simulink model "IEEE24bus"  (R2019b)
settings: Solver=VariableStepAuto  StartTime=0.0  StopTime=100  RelTol=1e-3
values from neighbouring files (symbols this model uses):
  C_b = 1/(w_b*Z_b)    (= 5.01433343075e-06)    [IEEE24_bus.m]
  Exc = [ 011	0	 200	0.02	1.12   0.5   0	0       0       0       0       0 ... (first row only)    [IEEE24_bus.m]
  G_data = [ 011	15.8 138	2.8	0.2     2.7	1.5     0.3     7.5     0.25	0.04	0.85	0.85	0.25	0.12	0 ... (first row only)    [IEEE24_bus.m]
  H011 = 4    [IEEE24_bus.m]
  H012 = 4    [IEEE24_bus.m]
  H013 = 4    [IEEE24_bus.m]
  H021 = 4    [IEEE24_bus.m]
  H022 = 4    [IEEE24_bus.m]
  H023 = 4    [IEEE24_bus.m]
  H024 = 4    [IEEE24_bus.m]
  H025 = 4    [IEEE24_bus.m]
  H026 = 4    [IEEE24_bus.m]
  H131 = 4    [IEEE24_bus.m]
  H132 = 4    [IEEE24_bus.m]
  H133 = 4    [IEEE24_bus.m]
  H134 = 4    [IEEE24_bus.m]
  H135 = 4    [IEEE24_bus.m]
  H151 = 4    [IEEE24_bus.m]
  H152 = 4    [IEEE24_bus.m]
  H153 = 4    [IEEE24_bus.m]
  H154 = 4    [IEEE24_bus.m]
  H161 = 4    [IEEE24_bus.m]
  H181 = 3.25    [IEEE24_bus.m]
  H211 = 4    [IEEE24_bus.m]
  H212 = 4    [IEEE24_bus.m]
  H213 = 4    [IEEE24_bus.m]
  H215 = 4    [IEEE24_bus.m]
  H216 = 4    [IEEE24_bus.m]
  H221 = 3.25    [IEEE24_bus.m]
  H231 = 4    [IEEE24_bus.m]
  H232 = 4    [IEEE24_bus.m]
  H233 = 4    [IEEE24_bus.m]
  H234 = 4    [IEEE24_bus.m]
  H235 = 4    [IEEE24_bus.m]
  L_b = Z_b/w_b    (= 1.40321608159)    [IEEE24_bus.m]
  PSSMODEL = 1    [IEEE24_bus.m]    (also in IEEE24bus_simplified_benchmark.m)
  Z_b = (V_b^2)/S_b    (= 529)    [IEEE24_bus.m]
undefined symbols (not defined in the file or in its folder): D1, Delta
libraries: powerlib x258, sps_avr x33, microgridLibrary x6
(part 4 of 6)

== system IEEE24bus/151 ==
  151 : powerlib/Machines/Synchronous Machine pu Standard  PresetModel=No  MechanicalLoad=Mechanical power Pm  ShowDetailedParameters=on  RotorType=Round  Units=per unit standard parameters  MeasurementBus=off  NominalParameters="[G_data(16,2)*1E6  G_data(16,3)*1E3  60]"  Reactances1=[G_data(16,6),G_data(16,8),G_data(16,10),G_data(16,7),G_data(16,12),G_data(16,14),G_data(16,5)]  Reactances2=[G_data(6,6),G_data(6,8),G_data(6,10),G_data(6,7),G_data(6,12),G_data(6,14),G_data(6,5)]  dAxisTimeConstants=Open-circuit  qAxisTimeConstants=Open-circuit  TimeConstants1="[G_data(6,9)  G_data(6,11)  G_data(6,13)  G_data(6,15)]"  TimeConstants2="[G_data(16,9)  G_data(16,11)  G_data(16,13)  G_data(16,15)]"  TimeConstants3="[  5.9  0.033  0.023  ]"  TimeConstants4=[ 8.0, 0.03, 0.3371, 0.0295 ]  TimeConstants5=[ 1.01, 0.053, 0.1 ]  TimeConstants6=[ 1.3201, 0.023, 1.0, 0.07 ]  TimeConstants7="[  1.01  0.053  0.051266  ]"  TimeConstants8=[ 1.3201, 0.0231, 0.3371, 0.0295 ]  StatorResistance=0  Mechanical="[ H151 0  4 ]"  PolePairs=4  InitialConditions=[0 -49.0871 0.832503 0.832503 0.832503 -10.6328 -130.633 109.367 2.39024]  SetSaturation=off  Saturation=[0.6404,0.7127,0.8441,0.9214,0.9956,1.082,1.19,1.316,1.457;0.7,0.7698,0.8872,0.9466,0.9969,1.046,1.1,1.151,1.201]  LoadFlowParameters=[1 3330000000 20000 0 0]  TsPowergui=0  TsBlock=-1  IterativeModel=Forward Euler  IterativeDiscreteModel=Trapezoidal non iterative  BusType=PV  Pref=G_data(16,2)*1e6  Qref=0  Qmin=-inf  Qmax=inf  PLF=0  QLF=0
      settings: SourceProductName=Simscape Power Systems
  AC4A Excitation System 151 : sps_avr/AC4A Excitation System  Tr=Exc(16,2)  KaTa="[Exc(16,3)   Exc(16,4)]"  VIminmax=[-10 10]  VRminmax=[-4.53 5.64]  TbTc="[Exc(16,5)  Exc(16,6)]"  Kc=0  v0=[1 2.3902]  TsBlock=0
      link override Model/Low Pass Filter 1//(Tr.s+1): Y0=Vt0  U0=Vt0
      settings: SourceProductName=Simscape Power Systems  SourceProductBaseCode=PS
  Bus Selector1 : BusSelector  OutputSignals="Mechanical.Rotor speed  wm  (pu),Output active power   Peo (pu),Mechanical.Rotor speed deviation  dw (pu),Mechanical.Rotor angle deviation  d_theta (rad),Mechanical.Rotor mechanical angle  theta (deg),dq0 components.Stator voltage  vd (pu),dq0 components.Stator voltage  vq (pu),dq0 components.Field current  ifd (pu),Output reactive power  Qeo (pu)"
  Complex to Magnitude-Angle : ComplexToMagnitudeAngle  Output=Magnitude
  "Delta Pa PSS 151 " : powerlib/Machines/Generic Power System Stabilizer  Tsensor=15e-3  K=2.5*1.25  Twashout=1  Tleadlag1=[60e-3 1]  Tleadlag2=[0 0]  VSlimits=[-0.15 0.15]  Vinit=0  Plot_On=off  MagdB_On=on  FreqRange=logspace(-2,2,500)
      settings: SourceProductName=Simscape Power Systems  SourceProductBaseCode=PS
  "Delta w PSS (Kundur) 151 " : powerlib/Machines/Generic Power System Stabilizer  Tsensor=15e-3  K=30  Twashout=10  Tleadlag1=[50e-3 20e-3]  Tleadlag2=[3 5.4]  VSlimits=[-0.15 0.15]  Vinit=0  Plot_On=off  MagdB_On=on  FreqRange=logspace(-2,2,500)
      settings: SourceProductName=Simscape Power Systems  SourceProductBaseCode=PS
  MB-PSS  151 : powerlib/Machines/Multi-Band Power System Stabilizer  OperationMode=Simplified settings  Kg=1  GL=[0.1 10]  GI="[1  10]"  GH="[13  120]"  GLd=[66 66 9.4]  TcLF=[1.667 2 0 0 0 0 2 2.4 0 0 0 0 1 1]  GId=[66 66 47.6]  TcIF=[1 1 0.25 0.3 0 0 1 1 0.3 0.36 0 0 0 0]  GHd=[66 66 233]  TcHF="[0.01 0.012 0 0 0 0  0.012 0.0144 0 0 0 0 1 1]"  LIM=[.075 .15 .15 .15]  Plot_On=off  MagdB_On=off  FreqRange=logspace(-2,2,500)
      settings: SourceProductName=Simscape Power Systems  SourceProductBaseCode=PS
  Multiport Switch1 : MultiPortSwitch  Inputs=4  InputSameDT=on
  PSS model3 : Constant  Value=0
  PSS model4 : Constant
  Pref : Constant
  Real-Imag to Complex : RealImagToComplex
  STG 151 : powerlib/Machines/Steam Turbine and Governor  gentype=Tandem-compound (single mass)  reg1="[ 1  0.05    0 ]"  reg2="[ 0.001  0.15 ]"  reg3="[ -0.1  0.1  0  4.496 ]"  N=3600  turb1="[ 0  10   3.3   0.5   ]"  turb2="[   0   0.36    0.36   0.28   ]"  HA="[ 0.046  1.430  1.465   0.192 ]"  KA="[ 90.44  53.88  64.59   62.94  ]"  DA="[ 0.0115  0.3575  0.3663   0.0137  ]"  ini1=0.9  ini2=[0.779316,-31.4247]
      settings: SourceProductName=Simscape Power Systems  SourceProductBaseCode=PS
  Sum2 : Sum  SaturateOnIntegerOverflow=on  InputSameDT=on  OutDataTypeStr=Inherit: Same as first input
  Sum3 : Sum  Inputs=-+  SaturateOnIntegerOverflow=on  InputSameDT=on  OutDataTypeStr=Inherit: Same as first input
  Terminator1 : Terminator
  Terminator2 : Terminator
  Terminator3 : Terminator
  Vref151 : Constant
  wref : Constant
  A : PMIOPort  Side=Left
  B : PMIOPort  Port=2  Side=Left
  C : PMIOPort  Port=3  Side=Left
  tag scope: EFD151=global, Pa151=global, Pe151=global, Pm151=global, Q151=global, Vt151=global, d_theta151=global, pss151=global, theta151=global, w151=global
  wires:
  Bus Selector1/7 -> Real-Imag to Complex/2  "<Stator voltage  vq (pu)>"
  Bus Selector1/6 -> Real-Imag to Complex/1  "<Stator voltage  vd (pu)>"
  wref/1 -> STG 151/1
  Vref151/1 -> AC4A Excitation System 151/1
  Bus Selector1/4 -> [d_theta151], STG 151/4  "<Rotor angle deviation  d_theta (rad)>"
  151/1 -> Bus Selector1/1, [M151]
  Bus Selector1/1 -> [w151], STG 151/3  "<Rotor speed  wm  (pu)>"
  Bus Selector1/3 -> "Delta w PSS (Kundur) 151 "/1, MB-PSS  151/1  "<Rotor speed deviation  dw (pu)>"
  Real-Imag to Complex/1 -> Complex to Magnitude-Angle/1
  Complex to Magnitude-Angle/1 -> AC4A Excitation System 151/2, [Vt151]
  AC4A Excitation System 151/1 -> 151/2, [EFD151]
  Multiport Switch1/1 -> AC4A Excitation System 151/4, [pss151]
  Bus Selector1/5 -> [theta151]  "<Rotor mechanical angle  theta (deg)>"
  Bus Selector1/2 -> [Pe151]  "<Output active power   Peo (pu)>"
  Bus Selector1/8 -> AC4A Excitation System 151/3  "<Field current  ifd (pu)>"
  STG 151/4 -> [Pm151], 151/1
  Pref/1 -> STG 151/2
  Bus Selector1/9 -> [Q151]  "<Output reactive power  Qeo (pu)>"
  PSS model4/1 -> Sum2/2
  Sum2/1 -> Multiport Switch1/1
  [PSSmodel] -> Sum2/1
  PSS model3/1 -> Multiport Switch1/2
  Sum3/1 -> [Pa151], "Delta Pa PSS 151 "/1  "Pm-Pe"
  "Delta Pa PSS 151 "/1 -> Multiport Switch1/5
  "Delta w PSS (Kundur) 151 "/1 -> Multiport Switch1/4
  [Pm151] -> Sum3/2
  [Pe151] -> Sum3/1
  MB-PSS  151/1 -> Multiport Switch1/3
  STG 151/1 -> Terminator3/1
  STG 151/2 -> Terminator1/1
  STG 151/3 -> Terminator2/1
  connections:
  151/RConn1 -- A/RConn1
  151/RConn2 -- B/RConn1
  151/RConn3 -- C/RConn1

== system IEEE24bus/152 ==
  152 : powerlib/Machines/Synchronous Machine pu Standard  PresetModel=No  MechanicalLoad=Mechanical power Pm  ShowDetailedParameters=on  RotorType=Round  Units=per unit standard parameters  MeasurementBus=off  NominalParameters="[310*1E6  G_data(17,3)*1E3  60]"  Reactances1=[G_data(17,6),G_data(17,8),G_data(17,10),G_data(17,7),G_data(17,12),G_data(17,14),G_data(17,5)]  Reactances2=[G_data(6,6),G_data(6,8),G_data(6,10),G_data(6,7),G_data(6,12),G_data(6,14),G_data(6,5)]  dAxisTimeConstants=Open-circuit  qAxisTimeConstants=Open-circuit  TimeConstants1="[G_data(6,9)  G_data(6,11)  G_data(6,13)  G_data(6,15)]"  TimeConstants2="[G_data(17,9)  G_data(17,11)  G_data(17,13)  G_data(17,15)]"  TimeConstants3="[  5.9  0.033  0.023  ]"  TimeConstants4=[ 8.0, 0.03, 0.3371, 0.0295 ]  TimeConstants5=[ 1.01, 0.053, 0.1 ]  TimeConstants6=[ 1.3201, 0.023, 1.0, 0.07 ]  TimeConstants7="[  1.01  0.053  0.051266  ]"  TimeConstants8=[ 1.3201, 0.0231, 0.3371, 0.0295 ]  StatorResistance=0  Mechanical="[ H152 0  4 ]"  PolePairs=4  InitialConditions=[0 -49.0871 0.832503 0.832503 0.832503 -10.6328 -130.633 109.367 2.39024]  SetSaturation=off  Saturation=[0.6404,0.7127,0.8441,0.9214,0.9956,1.082,1.19,1.316,1.457;0.7,0.7698,0.8872,0.9466,0.9969,1.046,1.1,1.151,1.201]  LoadFlowParameters=[1 3330000000 20000 0 0]  TsPowergui=0  TsBlock=-1  IterativeModel=Forward Euler  IterativeDiscreteModel=Trapezoidal non iterative  BusType=PV  Pref=310*1e6  Qref=0  Qmin=-inf  Qmax=inf  PLF=0  QLF=0
      settings: SourceProductName=Simscape Power Systems
  AC4A Excitation System 152 : sps_avr/AC4A Excitation System  Tr=Exc(17,2)  KaTa="[Exc(17,3)   Exc(17,4)]"  VIminmax=[-10 10]  VRminmax=[-4.53 5.64]  TbTc="[Exc(17,5)  Exc(17,6)]"  Kc=0  v0=[1 2.3902]  TsBlock=0
      link override Model/Low Pass Filter 1//(Tr.s+1): Y0=Vt0  U0=Vt0
      settings: SourceProductName=Simscape Power Systems  SourceProductBaseCode=PS
  Bus Selector1 : BusSelector  OutputSignals="Mechanical.Rotor speed  wm  (pu),Output active power   Peo (pu),Mechanical.Rotor speed deviation  dw (pu),Mechanical.Rotor angle deviation  d_theta (rad),Mechanical.Rotor mechanical angle  theta (deg),dq0 components.Stator voltage  vd (pu),dq0 components.Stator voltage  vq (pu),dq0 components.Field current  ifd (pu),Output reactive power  Qeo (pu)"
  Complex to Magnitude-Angle : ComplexToMagnitudeAngle  Output=Magnitude
  "Delta Pa PSS 152 " : powerlib/Machines/Generic Power System Stabilizer  Tsensor=15e-3  K=2.5*1.25  Twashout=1  Tleadlag1=[60e-3 1]  Tleadlag2=[0 0]  VSlimits=[-0.15 0.15]  Vinit=0  Plot_On=off  MagdB_On=on  FreqRange=logspace(-2,2,500)
      settings: SourceProductName=Simscape Power Systems  SourceProductBaseCode=PS
  "Delta w PSS (Kundur) 152 " : powerlib/Machines/Generic Power System Stabilizer  Tsensor=15e-3  K=30  Twashout=10  Tleadlag1=[50e-3 20e-3]  Tleadlag2=[3 5.4]  VSlimits=[-0.15 0.15]  Vinit=0  Plot_On=off  MagdB_On=on  FreqRange=logspace(-2,2,500)
      settings: SourceProductName=Simscape Power Systems  SourceProductBaseCode=PS
  MB-PSS  152 : powerlib/Machines/Multi-Band Power System Stabilizer  OperationMode=Simplified settings  Kg=1  GL=[0.1 10]  GI="[1  10]"  GH="[13  120]"  GLd=[66 66 9.4]  TcLF=[1.667 2 0 0 0 0 2 2.4 0 0 0 0 1 1]  GId=[66 66 47.6]  TcIF=[1 1 0.25 0.3 0 0 1 1 0.3 0.36 0 0 0 0]  GHd=[66 66 233]  TcHF="[0.01 0.012 0 0 0 0  0.012 0.0144 0 0 0 0 1 1]"  LIM=[.075 .15 .15 .15]  Plot_On=off  MagdB_On=off  FreqRange=logspace(-2,2,500)
      settings: SourceProductName=Simscape Power Systems  SourceProductBaseCode=PS
  Multiport Switch1 : MultiPortSwitch  Inputs=4  InputSameDT=on
  PSS model3 : Constant  Value=0
  PSS model4 : Constant
  Pref : Constant
  Real-Imag to Complex : RealImagToComplex
  STG 152 : powerlib/Machines/Steam Turbine and Governor  gentype=Tandem-compound (single mass)  reg1="[ 1  0.05    0 ]"  reg2="[ 0.001  0.15 ]"  reg3="[ -0.1  0.1  0  4.496 ]"  N=3600  turb1="[ 0  10   3.3   0.5   ]"  turb2="[   0   0.36    0.36   0.28   ]"  HA="[ 0.046  1.430  1.465   0.192 ]"  KA="[ 90.44  53.88  64.59   62.94  ]"  DA="[ 0.0115  0.3575  0.3663   0.0137  ]"  ini1=1  ini2=[0.779316,-31.4247]
      settings: SourceProductName=Simscape Power Systems  SourceProductBaseCode=PS
  Sum2 : Sum  SaturateOnIntegerOverflow=on  InputSameDT=on  OutDataTypeStr=Inherit: Same as first input
  Sum3 : Sum  Inputs=-+  SaturateOnIntegerOverflow=on  InputSameDT=on  OutDataTypeStr=Inherit: Same as first input
  Terminator1 : Terminator
  Terminator2 : Terminator
  Terminator3 : Terminator
  Vref15 : Constant
  wref : Constant
  A : PMIOPort  Side=Left
  B : PMIOPort  Port=2  Side=Left
  C : PMIOPort  Port=3  Side=Left
  tag scope: EFD152=global, Pa152=global, Pe152=global, Pm152=global, Q152=global, Vt152=global, d_theta152=global, pss152=global, theta152=global, w152=global
  wires:
  Bus Selector1/7 -> Real-Imag to Complex/2  "<Stator voltage  vq (pu)>"
  Bus Selector1/6 -> Real-Imag to Complex/1  "<Stator voltage  vd (pu)>"
  wref/1 -> STG 152/1
  Vref15/1 -> AC4A Excitation System 152/1
  Bus Selector1/4 -> [d_theta152], STG 152/4  "<Rotor angle deviation  d_theta (rad)>"
  152/1 -> Bus Selector1/1, [M152]
  Bus Selector1/1 -> [w152], STG 152/3  "<Rotor speed  wm  (pu)>"
  Bus Selector1/3 -> "Delta w PSS (Kundur) 152 "/1, MB-PSS  152/1  "<Rotor speed deviation  dw (pu)>"
  Real-Imag to Complex/1 -> Complex to Magnitude-Angle/1
  Complex to Magnitude-Angle/1 -> AC4A Excitation System 152/2, [Vt152]
  AC4A Excitation System 152/1 -> 152/2, [EFD152]
  Multiport Switch1/1 -> AC4A Excitation System 152/4, [pss152]
  Bus Selector1/5 -> [theta152]  "<Rotor mechanical angle  theta (deg)>"
  Bus Selector1/2 -> [Pe152]  "<Output active power   Peo (pu)>"
  Bus Selector1/8 -> AC4A Excitation System 152/3  "<Field current  ifd (pu)>"
  STG 152/4 -> [Pm152], 152/1
  Pref/1 -> STG 152/2
  Bus Selector1/9 -> [Q152]  "<Output reactive power  Qeo (pu)>"
  PSS model4/1 -> Sum2/2
  Sum2/1 -> Multiport Switch1/1
  [PSSmodel] -> Sum2/1
  PSS model3/1 -> Multiport Switch1/2
  Sum3/1 -> [Pa152], "Delta Pa PSS 152 "/1  "Pm-Pe"
  "Delta Pa PSS 152 "/1 -> Multiport Switch1/5
  "Delta w PSS (Kundur) 152 "/1 -> Multiport Switch1/4
  [Pm152] -> Sum3/2
  [Pe152] -> Sum3/1
  MB-PSS  152/1 -> Multiport Switch1/3
  STG 152/1 -> Terminator3/1
  STG 152/2 -> Terminator1/1
  STG 152/3 -> Terminator2/1
  connections:
  152/RConn1 -- A/RConn1
  152/RConn2 -- B/RConn1
  152/RConn3 -- C/RConn1

== system IEEE24bus/153 ==
  15 : powerlib/Machines/Synchronous Machine pu Standard  PresetModel=No  MechanicalLoad=Mechanical power Pm  ShowDetailedParameters=on  RotorType=Round  Units=per unit standard parameters  MeasurementBus=off  NominalParameters="[G_data(18,2)*1E6  G_data(18,3)*1E3  60]"  Reactances1=[G_data(18,6),G_data(18,8),G_data(18,10),G_data(18,7),G_data(18,12),G_data(18,14),G_data(18,5)]  Reactances2=[G_data(6,6),G_data(6,8),G_data(6,10),G_data(6,7),G_data(6,12),G_data(6,14),G_data(6,5)]  dAxisTimeConstants=Open-circuit  qAxisTimeConstants=Open-circuit  TimeConstants1="[G_data(6,9)  G_data(6,11)  G_data(6,13)  G_data(6,15)]"  TimeConstants2="[G_data(18,9)  G_data(18,11)  G_data(18,13)  G_data(18,15)]"  TimeConstants3="[  5.9  0.033  0.023  ]"  TimeConstants4=[ 8.0, 0.03, 0.3371, 0.0295 ]  TimeConstants5=[ 1.01, 0.053, 0.1 ]  TimeConstants6=[ 1.3201, 0.023, 1.0, 0.07 ]  TimeConstants7="[  1.01  0.053  0.051266  ]"  TimeConstants8=[ 1.3201, 0.0231, 0.3371, 0.0295 ]  StatorResistance=0  Mechanical="[ H153 0  4 ]"  PolePairs=4  InitialConditions=[0 -49.0871 0.832503 0.832503 0.832503 -10.6328 -130.633 109.367 2.39024]  SetSaturation=off  Saturation=[0.6404,0.7127,0.8441,0.9214,0.9956,1.082,1.19,1.316,1.457;0.7,0.7698,0.8872,0.9466,0.9969,1.046,1.1,1.151,1.201]  LoadFlowParameters=[1 3330000000 20000 0 0]  TsPowergui=0  TsBlock=-1  IterativeModel=Forward Euler  IterativeDiscreteModel=Trapezoidal non iterative  BusType=PV  Pref=G_data(18,2)*1e6  Qref=0  Qmin=-inf  Qmax=inf  PLF=0  QLF=0
      settings: SourceProductName=Simscape Power Systems
  AC4A Excitation System 153 : sps_avr/AC4A Excitation System  Tr=Exc(18,2)  KaTa="[Exc(18,3)   Exc(18,4)]"  VIminmax=[-10 10]  VRminmax=[-4.53 5.64]  TbTc="[Exc(18,5)  Exc(18,6)]"  Kc=0  v0=[1 2.3902]  TsBlock=0
      link override Model/Low Pass Filter 1//(Tr.s+1): Y0=Vt0  U0=Vt0
      settings: SourceProductName=Simscape Power Systems  SourceProductBaseCode=PS
  Bus Selector1 : BusSelector  OutputSignals="Mechanical.Rotor speed  wm  (pu),Output active power   Peo (pu),Mechanical.Rotor speed deviation  dw (pu),Mechanical.Rotor angle deviation  d_theta (rad),Mechanical.Rotor mechanical angle  theta (deg),dq0 components.Stator voltage  vd (pu),dq0 components.Stator voltage  vq (pu),dq0 components.Field current  ifd (pu),Output reactive power  Qeo (pu)"
  Complex to Magnitude-Angle : ComplexToMagnitudeAngle  Output=Magnitude
  "Delta Pa PSS 153 " : powerlib/Machines/Generic Power System Stabilizer  Tsensor=15e-3  K=2.5*1.25  Twashout=1  Tleadlag1=[60e-3 1]  Tleadlag2=[0 0]  VSlimits=[-0.15 0.15]  Vinit=0  Plot_On=off  MagdB_On=on  FreqRange=logspace(-2,2,500)
      settings: SourceProductName=Simscape Power Systems  SourceProductBaseCode=PS
  "Delta w PSS (Kundur) 153 " : powerlib/Machines/Generic Power System Stabilizer  Tsensor=15e-3  K=30  Twashout=10  Tleadlag1=[50e-3 20e-3]  Tleadlag2=[3 5.4]  VSlimits=[-0.15 0.15]  Vinit=0  Plot_On=off  MagdB_On=on  FreqRange=logspace(-2,2,500)
      settings: SourceProductName=Simscape Power Systems  SourceProductBaseCode=PS
  MB-PSS  153 : powerlib/Machines/Multi-Band Power System Stabilizer  OperationMode=Simplified settings  Kg=1  GL=[0.1 10]  GI="[1  10]"  GH="[13  120]"  GLd=[66 66 9.4]  TcLF=[1.667 2 0 0 0 0 2 2.4 0 0 0 0 1 1]  GId=[66 66 47.6]  TcIF=[1 1 0.25 0.3 0 0 1 1 0.3 0.36 0 0 0 0]  GHd=[66 66 233]  TcHF="[0.01 0.012 0 0 0 0  0.012 0.0144 0 0 0 0 1 1]"  LIM=[.075 .15 .15 .15]  Plot_On=off  MagdB_On=off  FreqRange=logspace(-2,2,500)
      settings: SourceProductName=Simscape Power Systems  SourceProductBaseCode=PS
  Multiport Switch1 : MultiPortSwitch  Inputs=4  InputSameDT=on
  PSS model3 : Constant  Value=0
  PSS model4 : Constant
  Pref : Constant
  Real-Imag to Complex : RealImagToComplex
  STG 153 : powerlib/Machines/Steam Turbine and Governor  gentype=Tandem-compound (single mass)  reg1="[ 1  0.05    0 ]"  reg2="[ 0.001  0.15 ]"  reg3="[ -0.1  0.1  0  4.496 ]"  N=3600  turb1="[ 0  10   3.3   0.5   ]"  turb2="[   0   0.36    0.36   0.28   ]"  HA="[ 0.046  1.430  1.465   0.192 ]"  KA="[ 90.44  53.88  64.59   62.94  ]"  DA="[ 0.0115  0.3575  0.3663   0.0137  ]"  ini1=0.9  ini2=[0.779316,-31.4247]
      settings: SourceProductName=Simscape Power Systems  SourceProductBaseCode=PS
  Sum2 : Sum  SaturateOnIntegerOverflow=on  InputSameDT=on  OutDataTypeStr=Inherit: Same as first input
  Sum3 : Sum  Inputs=-+  SaturateOnIntegerOverflow=on  InputSameDT=on  OutDataTypeStr=Inherit: Same as first input
  Terminator1 : Terminator
  Terminator2 : Terminator
  Terminator3 : Terminator
  Vref153 : Constant
  wref : Constant
  A : PMIOPort  Side=Left
  B : PMIOPort  Port=2  Side=Left
  C : PMIOPort  Port=3  Side=Left
  tag scope: EFD153=global, Pa153=global, Pe153=global, Pm153=global, Q153=global, Vt153=global, d_theta153=global, pss153=global, theta153=global, w153=global
  wires:
  Bus Selector1/7 -> Real-Imag to Complex/2  "<Stator voltage  vq (pu)>"
  Bus Selector1/6 -> Real-Imag to Complex/1  "<Stator voltage  vd (pu)>"
  wref/1 -> STG 153/1
  Vref153/1 -> AC4A Excitation System 153/1
  Bus Selector1/4 -> [d_theta153], STG 153/4  "<Rotor angle deviation  d_theta (rad)>"
  15/1 -> Bus Selector1/1, [M153]
  Bus Selector1/1 -> [w153], STG 153/3  "<Rotor speed  wm  (pu)>"
  Bus Selector1/3 -> "Delta w PSS (Kundur) 153 "/1, MB-PSS  153/1  "<Rotor speed deviation  dw (pu)>"
  Real-Imag to Complex/1 -> Complex to Magnitude-Angle/1
  Complex to Magnitude-Angle/1 -> AC4A Excitation System 153/2, [Vt153]
  AC4A Excitation System 153/1 -> 15/2, [EFD153]
  Multiport Switch1/1 -> AC4A Excitation System 153/4, [pss153]
  Bus Selector1/5 -> [theta153]  "<Rotor mechanical angle  theta (deg)>"
  Bus Selector1/2 -> [Pe153]  "<Output active power   Peo (pu)>"
  Bus Selector1/8 -> AC4A Excitation System 153/3  "<Field current  ifd (pu)>"
  STG 153/4 -> [Pm153], 15/1
  Pref/1 -> STG 153/2
  Bus Selector1/9 -> [Q153]  "<Output reactive power  Qeo (pu)>"
  PSS model4/1 -> Sum2/2
  Sum2/1 -> Multiport Switch1/1
  [PSSmodel] -> Sum2/1
  PSS model3/1 -> Multiport Switch1/2
  Sum3/1 -> [Pa153], "Delta Pa PSS 153 "/1  "Pm-Pe"
  "Delta Pa PSS 153 "/1 -> Multiport Switch1/5
  "Delta w PSS (Kundur) 153 "/1 -> Multiport Switch1/4
  [Pm153] -> Sum3/2
  [Pe153] -> Sum3/1
  MB-PSS  153/1 -> Multiport Switch1/3
  STG 153/1 -> Terminator3/1
  STG 153/2 -> Terminator1/1
  STG 153/3 -> Terminator2/1
  connections:
  15/RConn1 -- A/RConn1
  15/RConn2 -- B/RConn1
  15/RConn3 -- C/RConn1

== system IEEE24bus/154 ==
  154 : powerlib/Machines/Synchronous Machine pu Standard  PresetModel=No  MechanicalLoad=Mechanical power Pm  ShowDetailedParameters=on  RotorType=Round  Units=per unit standard parameters  MeasurementBus=off  NominalParameters="[G_data(19,2)*1E6  G_data(19,3)*1E3  60]"  Reactances1=[G_data(19,6),G_data(19,8),G_data(19,10),G_data(19,7),G_data(19,12),G_data(19,14),G_data(19,5)]  Reactances2=[G_data(6,6),G_data(6,8),G_data(6,10),G_data(6,7),G_data(6,12),G_data(6,14),G_data(6,5)]  dAxisTimeConstants=Open-circuit  qAxisTimeConstants=Open-circuit  TimeConstants1="[G_data(6,9)  G_data(6,11)  G_data(6,13)  G_data(6,15)]"  TimeConstants2="[G_data(19,9)  G_data(19,11)  G_data(19,13)  G_data(19,15)]"  TimeConstants3="[  5.9  0.033  0.023  ]"  TimeConstants4=[ 8.0, 0.03, 0.3371, 0.0295 ]  TimeConstants5=[ 1.01, 0.053, 0.1 ]  TimeConstants6=[ 1.3201, 0.023, 1.0, 0.07 ]  TimeConstants7="[  1.01  0.053  0.051266  ]"  TimeConstants8=[ 1.3201, 0.0231, 0.3371, 0.0295 ]  StatorResistance=0  Mechanical="[ H154 0  4 ]"  PolePairs=4  InitialConditions=[0 -49.0871 0.832503 0.832503 0.832503 -10.6328 -130.633 109.367 2.39024]  SetSaturation=off  Saturation=[0.6404,0.7127,0.8441,0.9214,0.9956,1.082,1.19,1.316,1.457;0.7,0.7698,0.8872,0.9466,0.9969,1.046,1.1,1.151,1.201]  LoadFlowParameters=[1 3330000000 20000 0 0]  TsPowergui=0  TsBlock=-1  IterativeModel=Forward Euler  IterativeDiscreteModel=Trapezoidal non iterative  BusType=PV  Pref=G_data(19,2)*1e6  Qref=0  Qmin=-inf  Qmax=inf  PLF=0  QLF=0
      settings: SourceProductName=Simscape Power Systems
  AC4A Excitation System 154 : sps_avr/AC4A Excitation System  Tr=Exc(19,2)  KaTa="[Exc(19,3)   Exc(19,4)]"  VIminmax=[-10 10]  VRminmax=[-4.53 5.64]  TbTc="[Exc(19,5)  Exc(19,6)]"  Kc=0  v0=[1 2.3902]  TsBlock=0
      link override Model/Low Pass Filter 1//(Tr.s+1): Y0=Vt0  U0=Vt0
      settings: SourceProductName=Simscape Power Systems  SourceProductBaseCode=PS
  Bus Selector1 : BusSelector  OutputSignals="Mechanical.Rotor speed  wm  (pu),Output active power   Peo (pu),Mechanical.Rotor speed deviation  dw (pu),Mechanical.Rotor angle deviation  d_theta (rad),Mechanical.Rotor mechanical angle  theta (deg),dq0 components.Stator voltage  vd (pu),dq0 components.Stator voltage  vq (pu),dq0 components.Field current  ifd (pu),Output reactive power  Qeo (pu)"
  Complex to Magnitude-Angle : ComplexToMagnitudeAngle  Output=Magnitude
  "Delta Pa PSS 154 " : powerlib/Machines/Generic Power System Stabilizer  Tsensor=15e-3  K=2.5*1.25  Twashout=1  Tleadlag1=[60e-3 1]  Tleadlag2=[0 0]  VSlimits=[-0.15 0.15]  Vinit=0  Plot_On=off  MagdB_On=on  FreqRange=logspace(-2,2,500)
      settings: SourceProductName=Simscape Power Systems  SourceProductBaseCode=PS
  "Delta w PSS (Kundur) 154 " : powerlib/Machines/Generic Power System Stabilizer  Tsensor=15e-3  K=30  Twashout=10  Tleadlag1=[50e-3 20e-3]  Tleadlag2=[3 5.4]  VSlimits=[-0.15 0.15]  Vinit=0  Plot_On=off  MagdB_On=on  FreqRange=logspace(-2,2,500)
      settings: SourceProductName=Simscape Power Systems  SourceProductBaseCode=PS
  MB-PSS  154 : powerlib/Machines/Multi-Band Power System Stabilizer  OperationMode=Simplified settings  Kg=1  GL=[0.1 10]  GI="[1  10]"  GH="[13  120]"  GLd=[66 66 9.4]  TcLF=[1.667 2 0 0 0 0 2 2.4 0 0 0 0 1 1]  GId=[66 66 47.6]  TcIF=[1 1 0.25 0.3 0 0 1 1 0.3 0.36 0 0 0 0]  GHd=[66 66 233]  TcHF="[0.01 0.012 0 0 0 0  0.012 0.0144 0 0 0 0 1 1]"  LIM=[.075 .15 .15 .15]  Plot_On=off  MagdB_On=off  FreqRange=logspace(-2,2,500)
      settings: SourceProductName=Simscape Power Systems  SourceProductBaseCode=PS
  Multiport Switch1 : MultiPortSwitch  Inputs=4  InputSameDT=on
  PSS model3 : Constant  Value=0
  PSS model4 : Constant
  Pref : Constant
  Real-Imag to Complex : RealImagToComplex
  STG 154 : powerlib/Machines/Steam Turbine and Governor  gentype=Tandem-compound (single mass)  reg1="[ 1  0.05    0 ]"  reg2="[ 0.001  0.15 ]"  reg3="[ -0.1  0.1  0  4.496 ]"  N=3600  turb1="[ 0  10   3.3   0.5   ]"  turb2="[   0   0.36    0.36   0.28   ]"  HA="[ 0.046  1.430  1.465   0.192 ]"  KA="[ 90.44  53.88  64.59   62.94  ]"  DA="[ 0.0115  0.3575  0.3663   0.0137  ]"  ini1=0.95  ini2=[0.779316,-31.4247]
      settings: SourceProductName=Simscape Power Systems  SourceProductBaseCode=PS
  Sum2 : Sum  SaturateOnIntegerOverflow=on  InputSameDT=on  OutDataTypeStr=Inherit: Same as first input
  Sum3 : Sum  Inputs=-+  SaturateOnIntegerOverflow=on  InputSameDT=on  OutDataTypeStr=Inherit: Same as first input
  Terminator1 : Terminator
  Terminator2 : Terminator
  Terminator3 : Terminator
  Vref15 : Constant
  wref : Constant
  A : PMIOPort  Side=Left
  B : PMIOPort  Port=2  Side=Left
  C : PMIOPort  Port=3  Side=Left
  tag scope: EFD154=global, Pa154=global, Pe154=global, Pm154=global, Q154=global, Vt154=global, d_theta154=global, pss154=global, theta154=global, w154=global
  wires:
  Bus Selector1/7 -> Real-Imag to Complex/2  "<Stator voltage  vq (pu)>"
  Bus Selector1/6 -> Real-Imag to Complex/1  "<Stator voltage  vd (pu)>"
  wref/1 -> STG 154/1
  Vref15/1 -> AC4A Excitation System 154/1
  Bus Selector1/4 -> [d_theta154], STG 154/4  "<Rotor angle deviation  d_theta (rad)>"
  154/1 -> Bus Selector1/1, [M154]
  Bus Selector1/1 -> [w154], STG 154/3  "<Rotor speed  wm  (pu)>"
  Bus Selector1/3 -> "Delta w PSS (Kundur) 154 "/1, MB-PSS  154/1  "<Rotor speed deviation  dw (pu)>"
  Real-Imag to Complex/1 -> Complex to Magnitude-Angle/1
  Complex to Magnitude-Angle/1 -> AC4A Excitation System 154/2, [Vt154]
  AC4A Excitation System 154/1 -> 154/2, [EFD154]
  Multiport Switch1/1 -> AC4A Excitation System 154/4, [pss154]
  Bus Selector1/5 -> [theta154]  "<Rotor mechanical angle  theta (deg)>"
  Bus Selector1/2 -> [Pe154]  "<Output active power   Peo (pu)>"
  Bus Selector1/8 -> AC4A Excitation System 154/3  "<Field current  ifd (pu)>"
  STG 154/4 -> [Pm154], 154/1
  Pref/1 -> STG 154/2
  Bus Selector1/9 -> [Q154]  "<Output reactive power  Qeo (pu)>"
  PSS model4/1 -> Sum2/2
  Sum2/1 -> Multiport Switch1/1
  [PSSmodel] -> Sum2/1
  PSS model3/1 -> Multiport Switch1/2
  Sum3/1 -> [Pa154], "Delta Pa PSS 154 "/1  "Pm-Pe"
  "Delta Pa PSS 154 "/1 -> Multiport Switch1/5
  "Delta w PSS (Kundur) 154 "/1 -> Multiport Switch1/4
  [Pm154] -> Sum3/2
  [Pe154] -> Sum3/1
  MB-PSS  154/1 -> Multiport Switch1/3
  STG 154/1 -> Terminator3/1
  STG 154/2 -> Terminator1/1
  STG 154/3 -> Terminator2/1
  connections:
  154/RConn1 -- A/RConn1
  154/RConn2 -- B/RConn1
  154/RConn3 -- C/RConn1

== system IEEE24bus/161 ==
  161 : powerlib/Machines/Synchronous Machine pu Standard  PresetModel=No  MechanicalLoad=Mechanical power Pm  ShowDetailedParameters=on  RotorType=Round  Units=per unit standard parameters  MeasurementBus=off  NominalParameters="[55*1E6  G_data(20,3)*1E3  60]"  Reactances1=[G_data(20,6),G_data(20,8),G_data(20,10),G_data(20,7),G_data(20,12),G_data(20,14),G_data(20,5)]  Reactances2=[G_data(6,6),G_data(6,8),G_data(6,10),G_data(6,7),G_data(6,12),G_data(6,14),G_data(6,5)]  dAxisTimeConstants=Open-circuit  qAxisTimeConstants=Open-circuit  TimeConstants1="[G_data(6,9)  G_data(6,11)  G_data(6,13)  G_data(6,15)]"  TimeConstants2="[G_data(20,9)  G_data(20,11)  G_data(20,13)  G_data(20,15)]"  TimeConstants3="[  5.9  0.033  0.023  ]"  TimeConstants4=[ 8.0, 0.03, 0.3371, 0.0295 ]  TimeConstants5=[ 1.01, 0.053, 0.1 ]  TimeConstants6=[ 1.3201, 0.023, 1.0, 0.07 ]  TimeConstants7="[  1.01  0.053  0.051266  ]"  TimeConstants8=[ 1.3201, 0.0231, 0.3371, 0.0295 ]  StatorResistance=0  Mechanical="[ H161 0  4 ]"  PolePairs=4  InitialConditions=[0 -54.0575 0.856287 0.856287 0.856287 -21.9961 -141.996 98.0039 2.02634]  SetSaturation=off  Saturation=[0.6404,0.7127,0.8441,0.9214,0.9956,1.082,1.19,1.316,1.457;0.7,0.7698,0.8872,0.9466,0.9969,1.046,1.1,1.151,1.201]  LoadFlowParameters=[1 3330000000 20000 0 0]  TsPowergui=0  TsBlock=-1  IterativeModel=Forward Euler  IterativeDiscreteModel=Trapezoidal non iterative  BusType=PV  Pref=54.25*1e6  Qref=0  Qmin=-inf  Qmax=inf  PLF=0  QLF=0
      settings: SourceProductName=Simscape Power Systems
  AC4A Excitation System 161 : sps_avr/AC4A Excitation System  Tr=Exc(20,2)  KaTa="[Exc(20,3)   Exc(20,4)]"  VIminmax=[-10 10]  VRminmax=[-4.53 5.64]  TbTc="[Exc(20,5)  Exc(20,6)]"  Kc=0  v0=[1 2.3902]  TsBlock=0
      settings: SourceProductName=Simscape Power Systems  SourceProductBaseCode=PS
  Bus Selector1 : BusSelector  OutputSignals="Mechanical.Rotor speed  wm  (pu),Output active power   Peo (pu),Mechanical.Rotor speed deviation  dw (pu),Mechanical.Rotor angle deviation  d_theta (rad),Mechanical.Rotor mechanical angle  theta (deg),dq0 components.Stator voltage  vd (pu),dq0 components.Stator voltage  vq (pu),dq0 components.Field current  ifd (pu),Output reactive power  Qeo (pu)"
  Complex to Magnitude-Angle : ComplexToMagnitudeAngle  Output=Magnitude
  "Delta Pa PSS 161 " : powerlib/Machines/Generic Power System Stabilizer  Tsensor=15e-3  K=2.5*1.25  Twashout=1  Tleadlag1=[60e-3 1]  Tleadlag2=[0 0]  VSlimits=[-0.15 0.15]  Vinit=0  Plot_On=off  MagdB_On=on  FreqRange=logspace(-2,2,500)
      settings: SourceProductName=Simscape Power Systems  SourceProductBaseCode=PS
  "Delta w PSS (Kundur) 161 " : powerlib/Machines/Generic Power System Stabilizer  Tsensor=15e-3  K=30  Twashout=10  Tleadlag1=[50e-3 20e-3]  Tleadlag2=[3 5.4]  VSlimits=[-0.15 0.15]  Vinit=0  Plot_On=off  MagdB_On=on  FreqRange=logspace(-2,2,500)
      settings: SourceProductName=Simscape Power Systems  SourceProductBaseCode=PS
  MB-PSS  161 : powerlib/Machines/Multi-Band Power System Stabilizer  OperationMode=Simplified settings  Kg=1  GL=[0.1 10]  GI="[1  10]"  GH="[13  120]"  GLd=[66 66 9.4]  TcLF=[1.667 2 0 0 0 0 2 2.4 0 0 0 0 1 1]  GId=[66 66 47.6]  TcIF=[1 1 0.25 0.3 0 0 1 1 0.3 0.36 0 0 0 0]  GHd=[66 66 233]  TcHF="[0.01 0.012 0 0 0 0  0.012 0.0144 0 0 0 0 1 1]"  LIM=[.075 .15 .15 .15]  Plot_On=off  MagdB_On=off  FreqRange=logspace(-2,2,500)
      settings: SourceProductName=Simscape Power Systems  SourceProductBaseCode=PS
  Multiport Switch1 : MultiPortSwitch  Inputs=4  InputSameDT=on
  PSS model3 : Constant  Value=0
  PSS model4 : Constant
  Pref : Constant
  Real-Imag to Complex : RealImagToComplex
  STG 161 : powerlib/Machines/Steam Turbine and Governor  gentype=Tandem-compound (single mass)  reg1="[ 1  0.05    0 ]"  reg2="[ 0.001  0.15 ]"  reg3="[ -0.1  0.1  0  4.496 ]"  N=3600  turb1="[ 0  10   3.3   0.5   ]"  turb2="[   0   0.36    0.36   0.28   ]"  HA="[ 0.046  1.430  1.465   0.192 ]"  KA="[ 90.44  53.88  64.59   62.94  ]"  DA="[ 0.0115  0.3575  0.3663   0.0137  ]"  ini1=0.98  ini2=[0.779316,-31.4247]
      settings: SourceProductName=Simscape Power Systems  SourceProductBaseCode=PS
  Sum2 : Sum  SaturateOnIntegerOverflow=on  InputSameDT=on  OutDataTypeStr=Inherit: Same as first input
  Sum3 : Sum  Inputs=-+  SaturateOnIntegerOverflow=on  InputSameDT=on  OutDataTypeStr=Inherit: Same as first input
  Terminator1 : Terminator
  Terminator2 : Terminator
  Terminator3 : Terminator
  Vref16 : Constant
  wref : Constant
  A : PMIOPort  Side=Left
  B : PMIOPort  Port=2  Side=Left
  C : PMIOPort  Port=3  Side=Left
  tag scope: EFD161=global, Pa161=global, Pe161=global, Pm161=global, Q161=global, Vt161=global, d_theta161=global, pss161=global, theta161=global, w161=global
  wires:
  Bus Selector1/7 -> Real-Imag to Complex/2  "<Stator voltage  vq (pu)>"
  Bus Selector1/6 -> Real-Imag to Complex/1  "<Stator voltage  vd (pu)>"
  wref/1 -> STG 161/1
  Vref16/1 -> AC4A Excitation System 161/1
  Bus Selector1/4 -> [d_theta161], STG 161/4  "<Rotor angle deviation  d_theta (rad)>"
  161/1 -> Bus Selector1/1, [M161]
  Bus Selector1/1 -> [w161], STG 161/3  "<Rotor speed  wm  (pu)>"
  Bus Selector1/3 -> "Delta w PSS (Kundur) 161 "/1, MB-PSS  161/1  "<Rotor speed deviation  dw (pu)>"
  Real-Imag to Complex/1 -> Complex to Magnitude-Angle/1
  Complex to Magnitude-Angle/1 -> AC4A Excitation System 161/2, [Vt161]
  AC4A Excitation System 161/1 -> 161/2, [EFD161]
  Multiport Switch1/1 -> AC4A Excitation System 161/4, [pss161]
  Bus Selector1/5 -> [theta161]  "<Rotor mechanical angle  theta (deg)>"
  Bus Selector1/2 -> [Pe161]  "<Output active power   Peo (pu)>"
  Bus Selector1/8 -> AC4A Excitation System 161/3  "<Field current  ifd (pu)>"
  STG 161/4 -> [Pm161], 161/1
  Pref/1 -> STG 161/2
  Bus Selector1/9 -> [Q161]  "<Output reactive power  Qeo (pu)>"
  PSS model4/1 -> Sum2/2
  Sum2/1 -> Multiport Switch1/1
  [PSSmodel] -> Sum2/1
  PSS model3/1 -> Multiport Switch1/2
  Sum3/1 -> [Pa161], "Delta Pa PSS 161 "/1  "Pm-Pe"
  "Delta Pa PSS 161 "/1 -> Multiport Switch1/5
  "Delta w PSS (Kundur) 161 "/1 -> Multiport Switch1/4
  [Pm161] -> Sum3/2
  [Pe161] -> Sum3/1
  MB-PSS  161/1 -> Multiport Switch1/3
  STG 161/1 -> Terminator3/1
  STG 161/2 -> Terminator1/1
  STG 161/3 -> Terminator2/1
  connections:
  161/RConn1 -- A/RConn1
  161/RConn2 -- B/RConn1
  161/RConn3 -- C/RConn1

== system IEEE24bus/181 ==
  181 : powerlib/Machines/Synchronous Machine pu Standard  PresetModel=No  MechanicalLoad=Mechanical power Pm  ShowDetailedParameters=on  RotorType=Round  Units=per unit standard parameters  MeasurementBus=off  NominalParameters="[190*1E6  G_data(21,3)*1E3  60]"  Reactances1=[G_data(21,6),G_data(21,8),G_data(21,10),G_data(21,7),G_data(21,12),G_data(21,14),G_data(21,5)]  Reactances2=[G_data(6,6),G_data(6,8),G_data(6,10),G_data(6,7),G_data(6,12),G_data(6,14),G_data(6,5)]  dAxisTimeConstants=Open-circuit  qAxisTimeConstants=Open-circuit  TimeConstants1="[G_data(6,9)  G_data(6,11)  G_data(6,13)  G_data(6,15)]"  TimeConstants2="[G_data(21,9)  G_data(21,11)  G_data(21,13)  G_data(21,15)]"  TimeConstants3="[  5.9  0.033  0.023  ]"  TimeConstants4=[ 8.0, 0.03, 0.3371, 0.0295 ]  TimeConstants5=[ 1.01, 0.053, 0.1 ]  TimeConstants6=[ 1.3201, 0.023, 1.0, 0.07 ]  TimeConstants7="[  1.01  0.053  0.051266  ]"  TimeConstants8=[ 1.3201, 0.0231, 0.3371, 0.0295 ]  StatorResistance=0  Mechanical="[ H181 0  4 ]"  PolePairs=4  InitialConditions=[0 -49.0871 0.832503 0.832503 0.832503 -10.6328 -130.633 109.367 2.39024]  SetSaturation=off  Saturation=[0.6404,0.7127,0.8441,0.9214,0.9956,1.082,1.19,1.316,1.457;0.7,0.7698,0.8872,0.9466,0.9969,1.046,1.1,1.151,1.201]  LoadFlowParameters=[1 3330000000 20000 0 0]  TsPowergui=0  TsBlock=-1  IterativeModel=Forward Euler  IterativeDiscreteModel=Trapezoidal non iterative  BusType=PV  Pref=187.55*1e6  Qref=0  Qmin=-inf  Qmax=inf  PLF=0  QLF=0
      settings: SourceProductName=Simscape Power Systems
  AC4A Excitation System 181 : sps_avr/AC4A Excitation System  Tr=Exc(21,2)  KaTa="[Exc(21,3)   Exc(21,4)]"  VIminmax=[-10 10]  VRminmax=[-4.53 5.64]  TbTc="[Exc(21,5)  Exc(21,6)]"  Kc=0  v0=[1 2.3902]  TsBlock=0
      settings: SourceProductName=Simscape Power Systems  SourceProductBaseCode=PS
  Bus Selector1 : BusSelector  OutputSignals="Mechanical.Rotor speed  wm  (pu),Output active power   Peo (pu),Mechanical.Rotor speed deviation  dw (pu),Mechanical.Rotor angle deviation  d_theta (rad),Mechanical.Rotor mechanical angle  theta (deg),dq0 components.Stator voltage  vd (pu),dq0 components.Stator voltage  vq (pu),dq0 components.Field current  ifd (pu),Output reactive power  Qeo (pu)"
  Complex to Magnitude-Angle : ComplexToMagnitudeAngle  Output=Magnitude
  "Delta Pa PSS 181 " : powerlib/Machines/Generic Power System Stabilizer  Tsensor=15e-3  K=2.5*1.25  Twashout=1  Tleadlag1=[60e-3 1]  Tleadlag2=[0 0]  VSlimits=[-0.15 0.15]  Vinit=0  Plot_On=off  MagdB_On=on  FreqRange=logspace(-2,2,500)
      settings: SourceProductName=Simscape Power Systems  SourceProductBaseCode=PS
  "Delta w PSS (Kundur) 181 " : powerlib/Machines/Generic Power System Stabilizer  Tsensor=15e-3  K=30  Twashout=10  Tleadlag1=[50e-3 20e-3]  Tleadlag2=[3 5.4]  VSlimits=[-0.15 0.15]  Vinit=0  Plot_On=off  MagdB_On=on  FreqRange=logspace(-2,2,500)
      settings: SourceProductName=Simscape Power Systems  SourceProductBaseCode=PS
  MB-PSS  181 : powerlib/Machines/Multi-Band Power System Stabilizer  OperationMode=Simplified settings  Kg=1  GL=[0.1 10]  GI="[1  10]"  GH="[13  120]"  GLd=[66 66 9.4]  TcLF=[1.667 2 0 0 0 0 2 2.4 0 0 0 0 1 1]  GId=[66 66 47.6]  TcIF=[1 1 0.25 0.3 0 0 1 1 0.3 0.36 0 0 0 0]  GHd=[66 66 233]  TcHF="[0.01 0.012 0 0 0 0  0.012 0.0144 0 0 0 0 1 1]"  LIM=[.075 .15 .15 .15]  Plot_On=off  MagdB_On=off  FreqRange=logspace(-2,2,500)
      settings: SourceProductName=Simscape Power Systems  SourceProductBaseCode=PS
  Multiport Switch1 : MultiPortSwitch  Inputs=4  InputSameDT=on
  PSS model3 : Constant  Value=0
  PSS model4 : Constant
  Pref : Constant
  Real-Imag to Complex : RealImagToComplex
  STG 181 : powerlib/Machines/Steam Turbine and Governor  gentype=Tandem-compound (single mass)  reg1="[ 1  0.05    0 ]"  reg2="[ 0.001  0.15 ]"  reg3="[ -0.1  0.1  0  4.496 ]"  N=3600  turb1="[ 0  10   3.3   0.5   ]"  turb2="[   0   0.36    0.36   0.28   ]"  HA="[ 0.046  1.430  1.465   0.192 ]"  KA="[ 90.44  53.88  64.59   62.94  ]"  DA="[ 0.0115  0.3575  0.3663   0.0137  ]"  ini1=0.95  ini2=[0.779316,-31.4247]
      settings: SourceProductName=Simscape Power Systems  SourceProductBaseCode=PS
  Sum2 : Sum  SaturateOnIntegerOverflow=on  InputSameDT=on  OutDataTypeStr=Inherit: Same as first input
  Sum3 : Sum  Inputs=-+  SaturateOnIntegerOverflow=on  InputSameDT=on  OutDataTypeStr=Inherit: Same as first input
  Terminator1 : Terminator
  Terminator2 : Terminator
  Terminator3 : Terminator
  Vref181 : Constant
  wref : Constant
  A : PMIOPort  Side=Left
  B : PMIOPort  Port=2  Side=Left
  C : PMIOPort  Port=3  Side=Left
  tag scope: EFD181=global, Pa181=global, Pe181=global, Pm181=global, Q181=global, Vt181=global, d_theta181=global, pss181=global, theta181=global, w181=global
  wires:
  Bus Selector1/7 -> Real-Imag to Complex/2  "<Stator voltage  vq (pu)>"
  Bus Selector1/6 -> Real-Imag to Complex/1  "<Stator voltage  vd (pu)>"
  wref/1 -> STG 181/1
  Vref181/1 -> AC4A Excitation System 181/1
  Bus Selector1/4 -> [d_theta181], STG 181/4  "<Rotor angle deviation  d_theta (rad)>"
  181/1 -> Bus Selector1/1, [M181]
  Bus Selector1/1 -> [w181], STG 181/3  "<Rotor speed  wm  (pu)>"
  Bus Selector1/3 -> "Delta w PSS (Kundur) 181 "/1, MB-PSS  181/1  "<Rotor speed deviation  dw (pu)>"
  Real-Imag to Complex/1 -> Complex to Magnitude-Angle/1
  Complex to Magnitude-Angle/1 -> AC4A Excitation System 181/2, [Vt181]
  AC4A Excitation System 181/1 -> 181/2, [EFD181]
  Multiport Switch1/1 -> AC4A Excitation System 181/4, [pss181]
  Bus Selector1/5 -> [theta181]  "<Rotor mechanical angle  theta (deg)>"
  Bus Selector1/2 -> [Pe181]  "<Output active power   Peo (pu)>"
  Bus Selector1/8 -> AC4A Excitation System 181/3  "<Field current  ifd (pu)>"
  STG 181/4 -> [Pm181], 181/1
  Pref/1 -> STG 181/2
  Bus Selector1/9 -> [Q181]  "<Output reactive power  Qeo (pu)>"
  PSS model4/1 -> Sum2/2
  Sum2/1 -> Multiport Switch1/1
  [PSSmodel] -> Sum2/1
  PSS model3/1 -> Multiport Switch1/2
  Sum3/1 -> [Pa181], "Delta Pa PSS 181 "/1  "Pm-Pe"
  "Delta Pa PSS 181 "/1 -> Multiport Switch1/5
  "Delta w PSS (Kundur) 181 "/1 -> Multiport Switch1/4
  [Pm181] -> Sum3/2
  [Pe181] -> Sum3/1
  MB-PSS  181/1 -> Multiport Switch1/3
  STG 181/1 -> Terminator3/1
  STG 181/2 -> Terminator1/1
  STG 181/3 -> Terminator2/1
  connections:
  181/RConn1 -- A/RConn1
  181/RConn2 -- B/RConn1
  181/RConn3 -- C/RConn1

== system IEEE24bus/211 ==
  211 : powerlib/Machines/Synchronous Machine pu Standard  PresetModel=No  MechanicalLoad=Mechanical power Pm  ShowDetailedParameters=on  RotorType=Round  Units=per unit standard parameters  MeasurementBus=off  NominalParameters="[180*1E6  G_data(23,3)*1E3  60]"  Reactances1=[G_data(23,6),G_data(23,8),G_data(23,10),G_data(23,7),G_data(23,12),G_data(23,14),G_data(23,5)]  Reactances2=[G_data(6,6),G_data(6,8),G_data(6,10),G_data(6,7),G_data(6,12),G_data(6,14),G_data(6,5)]  dAxisTimeConstants=Open-circuit  qAxisTimeConstants=Open-circuit  TimeConstants1="[G_data(6,9)  G_data(6,11)  G_data(6,13)  G_data(6,15)]"  TimeConstants2="[G_data(23,9)  G_data(23,11)  G_data(23,13)  G_data(23,15)]"  TimeConstants3="[  5.9  0.033  0.023  ]"  TimeConstants4=[ 8.0, 0.03, 0.3371, 0.0295 ]  TimeConstants5=[ 1.01, 0.053, 0.1 ]  TimeConstants6=[ 1.3201, 0.023, 1.0, 0.07 ]  TimeConstants7="[  1.01  0.053  0.051266  ]"  TimeConstants8=[ 1.3201, 0.0231, 0.3371, 0.0295 ]  StatorResistance=0  Mechanical="[ H211 0  4 ]"  PolePairs=4  InitialConditions=[0 -49.0871 0.832503 0.832503 0.832503 -10.6328 -130.633 109.367 2.39024]  SetSaturation=off  Saturation=[0.6404,0.7127,0.8441,0.9214,0.9956,1.082,1.19,1.316,1.457;0.7,0.7698,0.8872,0.9466,0.9969,1.046,1.1,1.151,1.201]  LoadFlowParameters=[1 3330000000 20000 0 0]  TsPowergui=0  TsBlock=-1  IterativeModel=Forward Euler  IterativeDiscreteModel=Trapezoidal non iterative  BusType=PV  Pref=180*1e6  Qref=0  Qmin=-inf  Qmax=inf  PLF=0  QLF=0
      settings: SourceProductName=Simscape Power Systems
  AC4A Excitation System 211 : sps_avr/AC4A Excitation System  Tr=Exc(23,2)  KaTa="[Exc(23,3)   Exc(23,4)]"  VIminmax=[-10 10]  VRminmax=[-4.53 5.64]  TbTc="[Exc(23,5)  Exc(23,6)]"  Kc=0  v0=[1 2.3902]  TsBlock=0
      settings: SourceProductName=Simscape Power Systems  SourceProductBaseCode=PS
  Bus Selector1 : BusSelector  OutputSignals="Mechanical.Rotor speed  wm  (pu),Output active power   Peo (pu),Mechanical.Rotor speed deviation  dw (pu),Mechanical.Rotor angle deviation  d_theta (rad),Mechanical.Rotor mechanical angle  theta (deg),dq0 components.Stator voltage  vd (pu),dq0 components.Stator voltage  vq (pu),dq0 components.Field current  ifd (pu),Output reactive power  Qeo (pu)"
  Complex to Magnitude-Angle : ComplexToMagnitudeAngle  Output=Magnitude
  "Delta Pa PSS 211 " : powerlib/Machines/Generic Power System Stabilizer  Tsensor=15e-3  K=2.5*1.25  Twashout=1  Tleadlag1=[60e-3 1]  Tleadlag2=[0 0]  VSlimits=[-0.15 0.15]  Vinit=0  Plot_On=off  MagdB_On=on  FreqRange=logspace(-2,2,500)
      settings: SourceProductName=Simscape Power Systems  SourceProductBaseCode=PS
  "Delta w PSS (Kundur) 211 " : powerlib/Machines/Generic Power System Stabilizer  Tsensor=15e-3  K=30  Twashout=10  Tleadlag1=[50e-3 20e-3]  Tleadlag2=[3 5.4]  VSlimits=[-0.15 0.15]  Vinit=0  Plot_On=off  MagdB_On=on  FreqRange=logspace(-2,2,500)
      settings: SourceProductName=Simscape Power Systems  SourceProductBaseCode=PS
  MB-PSS  211 : powerlib/Machines/Multi-Band Power System Stabilizer  OperationMode=Simplified settings  Kg=1  GL=[0.1 10]  GI="[1  10]"  GH="[13  120]"  GLd=[66 66 9.4]  TcLF=[1.667 2 0 0 0 0 2 2.4 0 0 0 0 1 1]  GId=[66 66 47.6]  TcIF=[1 1 0.25 0.3 0 0 1 1 0.3 0.36 0 0 0 0]  GHd=[66 66 233]  TcHF="[0.01 0.012 0 0 0 0  0.012 0.0144 0 0 0 0 1 1]"  LIM=[.075 .15 .15 .15]  Plot_On=off  MagdB_On=off  FreqRange=logspace(-2,2,500)
      settings: SourceProductName=Simscape Power Systems  SourceProductBaseCode=PS
  Multiport Switch1 : MultiPortSwitch  Inputs=4  InputSameDT=on
  PSS model3 : Constant  Value=0
  PSS model4 : Constant
  Pref : Constant
  Real-Imag to Complex : RealImagToComplex
  STG 211 : powerlib/Machines/Steam Turbine and Governor  gentype=Tandem-compound (single mass)  reg1="[ 1  0.05    0 ]"  reg2="[ 0.001  0.15 ]"  reg3="[ -0.1  0.1  0  4.496 ]"  N=3600  turb1="[ 0  10   3.3   0.5   ]"  turb2="[   0   0.36    0.36   0.28   ]"  HA="[ 0.046  1.430  1.465   0.192 ]"  KA="[ 90.44  53.88  64.59   62.94  ]"  DA="[ 0.0115  0.3575  0.3663   0.0137  ]"  ini1=1  ini2=[0.779316,-31.4247]
      settings: SourceProductName=Simscape Power Systems  SourceProductBaseCode=PS
  Sum2 : Sum  SaturateOnIntegerOverflow=on  InputSameDT=on  OutDataTypeStr=Inherit: Same as first input
  Sum3 : Sum  Inputs=-+  SaturateOnIntegerOverflow=on  InputSameDT=on  OutDataTypeStr=Inherit: Same as first input
  Terminator1 : Terminator
  Terminator2 : Terminator
  Terminator3 : Terminator
  Vref21 : Constant
  wref : Constant
  A : PMIOPort  Side=Left
  B : PMIOPort  Port=2  Side=Left
  C : PMIOPort  Port=3  Side=Left
  tag scope: EFD211=global, Pa211=global, Pe211=global, Pm211=global, Q211=global, Vt211=global, d_theta211=global, pss211=global, theta211=global, w211=global
  wires:
  Bus Selector1/7 -> Real-Imag to Complex/2  "<Stator voltage  vq (pu)>"
  Bus Selector1/6 -> Real-Imag to Complex/1  "<Stator voltage  vd (pu)>"
  wref/1 -> STG 211/1
  Vref21/1 -> AC4A Excitation System 211/1
  Bus Selector1/4 -> [d_theta211], STG 211/4  "<Rotor angle deviation  d_theta (rad)>"
  211/1 -> Bus Selector1/1, [M211]
  Bus Selector1/1 -> [w211], STG 211/3  "<Rotor speed  wm  (pu)>"
  Bus Selector1/3 -> "Delta w PSS (Kundur) 211 "/1, MB-PSS  211/1  "<Rotor speed deviation  dw (pu)>"
  Real-Imag to Complex/1 -> Complex to Magnitude-Angle/1
  Complex to Magnitude-Angle/1 -> AC4A Excitation System 211/2, [Vt211]
  AC4A Excitation System 211/1 -> 211/2, [EFD211]
  Multiport Switch1/1 -> AC4A Excitation System 211/4, [pss211]
  Bus Selector1/5 -> [theta211]  "<Rotor mechanical angle  theta (deg)>"
  Bus Selector1/2 -> [Pe211]  "<Output active power   Peo (pu)>"
  Bus Selector1/8 -> AC4A Excitation System 211/3  "<Field current  ifd (pu)>"
  STG 211/4 -> [Pm211], 211/1
  Pref/1 -> STG 211/2
  Bus Selector1/9 -> [Q211]  "<Output reactive power  Qeo (pu)>"
  PSS model4/1 -> Sum2/2
  Sum2/1 -> Multiport Switch1/1
  [PSSmodel] -> Sum2/1
  PSS model3/1 -> Multiport Switch1/2
  Sum3/1 -> [Pa211], "Delta Pa PSS 211 "/1  "Pm-Pe"
  "Delta Pa PSS 211 "/1 -> Multiport Switch1/5
  "Delta w PSS (Kundur) 211 "/1 -> Multiport Switch1/4
  [Pm211] -> Sum3/2
  [Pe211] -> Sum3/1
  MB-PSS  211/1 -> Multiport Switch1/3
  STG 211/1 -> Terminator3/1
  STG 211/2 -> Terminator1/1
  STG 211/3 -> Terminator2/1
  connections:
  211/RConn1 -- A/RConn1
  211/RConn2 -- B/RConn1
  211/RConn3 -- C/RConn1
